simulink model "findmaxRaibert"  (R2014b)
settings: Solver=ode3  StartTime=0.0  StopTime=.25  FixedStep=.01  RelTol=1e-3
values from neighbouring files (symbols this model uses):
  alpha = alpha2.signals.values(end)    [BslipRaibert.m]
  k = 280    [BslipRaibert.m]
  xf = 0    [BslipRaibert.m]
  xinS = xd1.signals.values(end)    [BslipRaibert.m]
  xp = xd.signals.values(end)-(cos(alpha/180*pi)-xpp)    [BslipRaibert.m]
  yinS = yd1.signals.values(end)    [BslipRaibert.m]
  yp = yd.signals.values(end)    [BslipRaibert.m]
settings Model: Creator=hamidreza  LastModifiedBy=hamidreza

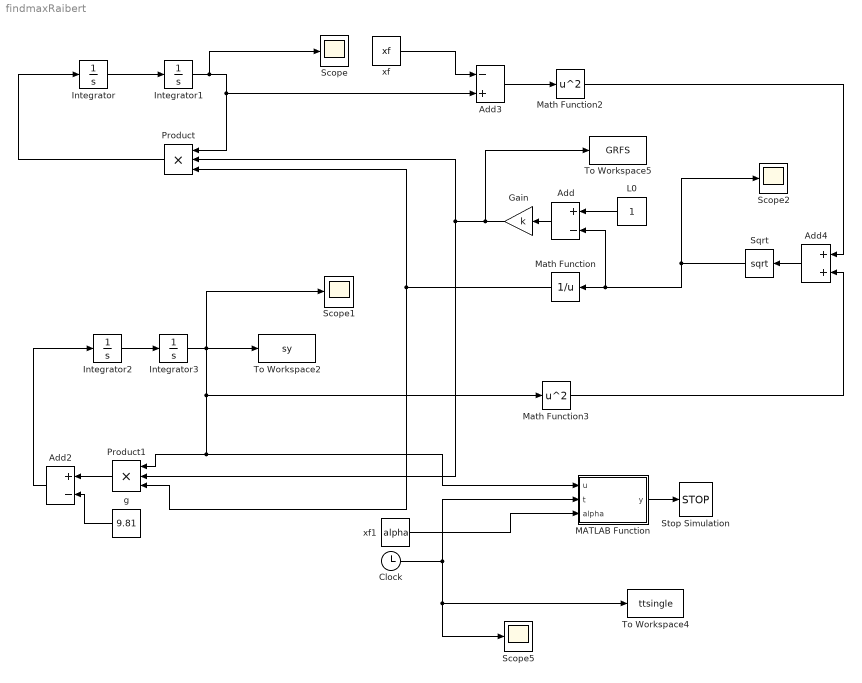
== system findmaxRaibert ==
  Add : Sum  Inputs=+-
  Add2 : Sum  Inputs=+-
  Add3 : Sum  Inputs=-+
  Add4 : Sum
  Clock : Clock
  Gain : Gain  Gain=k
  Integrator : Integrator  InitialCondition=xinS
  Integrator1 : Integrator  InitialCondition=xp
  Integrator2 : Integrator  InitialCondition=yinS
  Integrator3 : Integrator  InitialCondition=yp
  L0 : Constant
  MATLAB Function : MATLAB Function  TreatAsAtomicUnit=on
  Math Function : Math  Operator=reciprocal  SaturateOnIntegerOverflow=on
  Math Function2 : Math  Operator=square  SaturateOnIntegerOverflow=on
  Math Function3 : Math  Operator=square  SaturateOnIntegerOverflow=on
  Product : Product  Inputs=3
  Product1 : Product  Inputs=3
  Scope{,1..2,5} (4 alike) : Scope
      Scope settings: TimeRange=0.17  YMin=-0.102  YMax=-0.088
      Scope1 settings: TimeRange=0.11  YMin=0.965  YMax=0.98
      Scope2 settings: TimeRange=0.14  YMin=0.97  YMax=1.005  SaveName=ScopeData2
      Scope5 settings: TimeRange=0.14  YMin=0.97  YMax=1.005  SaveName=ScopeData5
  Sqrt : Sqrt  SaturateOnIntegerOverflow=on
  Stop Simulation : Stop
  To Workspace2 : ToWorkspace  VariableName=sy  SaveFormat=Structure With Time  SampleTime=-1
  To Workspace4 : ToWorkspace  VariableName=ttsingle  SampleTime=-1
      settings: Save2DSignal=2-D array (concatenate along first dimension)
  To Workspace5 : ToWorkspace  VariableName=GRFS  SaveFormat=Structure With Time  SampleTime=-1
      settings: Save2DSignal=2-D array (concatenate along first dimension)
  g : Constant  Value=9.81
  xf : Constant  Value=xf
  xf1 : Constant  Value=alpha
  wires:
  Integrator/1 -> Integrator1/1
  Product/1 -> Integrator/1
  Add/1 -> Gain/1
  Integrator2/1 -> Integrator3/1
  Product1/1 -> Add2/1
  g/1 -> Add2/2
  Add2/1 -> Integrator2/1
  xf/1 -> Add3/1
  Add3/1 -> Math Function2/1
  Math Function2/1 -> Add4/1
  Add4/1 -> Sqrt/1
  Sqrt/1 -> Add/2, Math Function/1, Scope2/1
  L0/1 -> Add/1
  Integrator3/1 -> Scope1/1, Product1/1, MATLAB Function/1(u), Math Function3/1, To Workspace2/1
  Clock/1 -> To Workspace4/1, Scope5/1, MATLAB Function/2(t)
  MATLAB Function/1(y) -> Stop Simulation/1
  Math Function3/1 -> Add4/2
  Gain/1 -> To Workspace5/1, Product1/2, Product/2
  Math Function/1 -> Product/3, Product1/3
  Integrator1/1 -> Scope/1, Add3/2, Product/1
  xf1/1 -> MATLAB Function/3(alpha)

== matlab function findmaxRaibert/MATLAB Function ==
  data: u input; y output; t input; alpha input
function y = fcn(u,t,alpha)
%#codegen

if and(u-sin(alpha/180*pi)<.001,t>.04)
    y=1;
else
    y=0;

end
